simulink model "sys_variations"  (R2016b)
settings: Solver=ode3  StartTime=0.0  StopTime=Tsim  FixedStep=Ts  RelTol=1e-3  EnableMultiTasking=on
undefined symbols (not defined in the file or in its folder): C_meas1, C_meas2, C_out1, C_out2, dist, K, Preal, Pref, ref, Tdist, Tref, xK0, xreal0, xref0
settings Model: Creator=Matti  LastModifiedBy=user
settings OptimizationCC: LifeSpan=inf
settings DebuggingCC: SFUnexpectedBacktrackingDiag=warning  SFNoUnconditionalDefaultTransitionDiag=warning  SFExecutionAtInitializationDiag=none
settings GRTTargetCC: TargetLangStandard=C89/C90 (ANSI)  GeneratePreprocessorConditionals=Disable all
settings ConfigComp: CovMetricSettings=dw  CovHtmlReporting=on  CovSaveCumulativeToWorkspaceVar=on  CovSaveSingleToWorkspaceVar=on  CovExternalEMLEnable=off

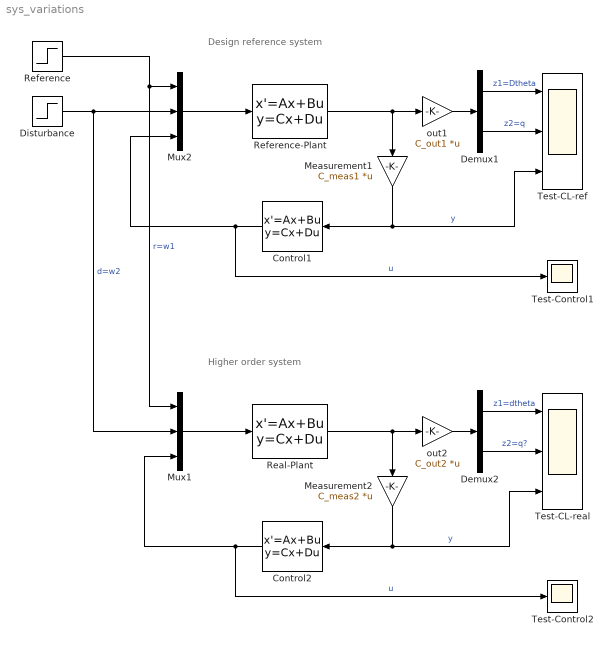
== system sys_variations ==
  note: Design reference system
  note: Higher order system
  Control1 : StateSpace  A=K.A  B=K.B  C=K.C  D=K.D  X0=xK0
  Control2 : StateSpace  A=K.A  B=K.B  C=K.C  D=K.D  X0=xK0
  Demux1 : Demux  Outputs=2
  Demux2 : Demux  Outputs=2
  Disturbance : Step  Time=Tdist  After=dist  SampleTime=0
  Measurement1 : Gain  Gain=C_meas1  Multiplication=Matrix(K*u)
  Measurement2 : Gain  Gain=C_meas2  Multiplication=Matrix(K*u)
  Mux1 : Mux  Inputs=3
  Mux2 : Mux  Inputs=3
  Real-Plant : StateSpace  A=Preal.A  B=Preal.B  C=Preal.C  D=Preal.D  X0=xreal0
  Reference : Step  Time=Tref  After=ref  SampleTime=0
  Reference-Plant : StateSpace  A=Pref.A  B=Pref.B  C=Pref.C  D=Pref.D  X0=xref0
  Test-CL-real : Scope  NumInputPorts=3
  Test-CL-ref : Scope  NumInputPorts=3
  Test-Control1 : Scope
  Test-Control2 : Scope
  out1 : Gain  Gain=C_out1  Multiplication=Matrix(K*u)
  out2 : Gain  Gain=C_out2  Multiplication=Matrix(K*u)
  wires:
  Disturbance/1 -> Mux1/2, Mux2/2  "d=w2"
  Measurement1/1 -> Test-CL-ref/3, Control1/1  "y"
  Reference-Plant/1 -> Measurement1/1, out1/1
  Control1/1 -> Test-Control1/1, Mux2/3  "u"
  Mux2/1 -> Reference-Plant/1
  Reference/1 -> Mux1/1, Mux2/1  "r=w1"
  Demux1/1 -> Test-CL-ref/1  "z1=Dtheta"
  out1/1 -> Demux1/1
  Demux1/2 -> Test-CL-ref/2  "z2=q"
  Measurement2/1 -> Control2/1, Test-CL-real/3  "y"
  Real-Plant/1 -> Measurement2/1, out2/1
  Control2/1 -> Test-Control2/1, Mux1/3  "u"
  Mux1/1 -> Real-Plant/1
  Demux2/1 -> Test-CL-real/1  "z1=dtheta"
  out2/1 -> Demux2/1
  Demux2/2 -> Test-CL-real/2  "z2=q?"
